simulink model "NN_EKF_Quadrotor_trajectory_control_p"  (Simulink 10.0)
settings: Solver=ode4  StartTime=0.0  StopTime=25  FixedStep=0.001  RelTol=1e-3  EnableMultiTasking=on
settings Model: Creator=Alireza  LastModifiedBy=7385281
settings DataIOCC: LimitDataPoints=on  SignalLoggingSaveFormat=ModelDataLogs
settings OptimizationCC: ExpressionDepthLimit=2147483647
settings DebuggingCC: SolverPrmCheckMsg=warning  FcnCallInpInsideContextMsg=warning  AllowSymbolicDim=off  StateNameClashWarn=warning
settings GRTTargetCC: GeneratePreprocessorConditionals=Disable all
settings ConfigComp: CovExternalEMLEnable=off

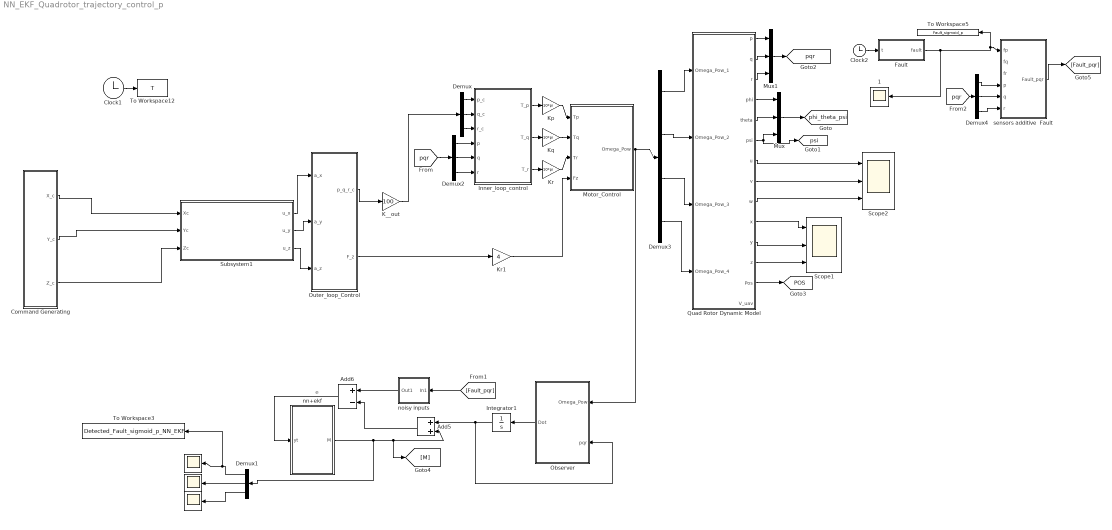
== system NN_EKF_Quadrotor_trajectory_control_p ==
  note: e
  "     " : Scope
  "      " : Scope
  "          " : Scope
  "     1" : Scope
  Add5 : Sum
  Add6 : Sum  Inputs=+-  OutDataTypeStr=Inherit: Same as accumulator
  Clock1 : Clock
  Clock2 : Clock
  Command Generating : Subsystem
  Demux{,1..2,4} (4 alike) : Demux  Outputs=3
  Demux3 : Demux
  Fault : MATLAB Function  TreatAsAtomicUnit=on
  Inner_loop_control : MATLAB Function  TreatAsAtomicUnit=on
  Integrator1 : Integrator  InitialCondition=[0.0001;0.0001;0.0001]
  K__out : Gain  Gain=100
  Kp : Gain  Gain=10*pi
  Kq : Gain  Gain=10*pi
  Kr : Gain  Gain=10*pi
  Kr1 : Gain  Gain=4
  Motor_Control : MATLAB Function  TreatAsAtomicUnit=on
  Mux : Mux  Inputs=3
  Mux1 : Mux  Inputs=3
  Observer : MATLAB Function  TreatAsAtomicUnit=on
  Outer_loop_Control : Subsystem
  Quad Rotor Dynamic Model : Subsystem
  Scope1 : Scope  NumInputPorts=3
  Scope2 : Scope  NumInputPorts=3
  Subsystem1 : Subsystem
  To Workspace12 : ToWorkspace  VariableName=T  SampleTime=-1
  To Workspace3 : ToWorkspace  VariableName=Detected_Fault_sigmoid_p_NN_EKF  SampleTime=-1
  To Workspace5 : ToWorkspace  VariableName=Fault_sigmoid_p  SampleTime=-1
  nn+ekf : Subsystem
  noisy inputs : Subsystem
  "sensors additive  Fault " : MATLAB Function  TreatAsAtomicUnit=on
  tag scope: POS=global, phi_theta_psi=global, pqr=global, psi=global
  wires:
  Quad Rotor Dynamic Model/4(phi) -> Mux/1
  Quad Rotor Dynamic Model/5(theta) -> Mux/2
  Quad Rotor Dynamic Model/6(psi) -> Mux/3, [psi]
  Mux/1 -> [phi_theta_psi]
  Inner_loop_control/1(T_p) -> Kp/1
  Inner_loop_control/2(T_q) -> Kq/1
  Inner_loop_control/3(T_r) -> Kr/1
  Quad Rotor Dynamic Model/1(p) -> Mux1/1
  Quad Rotor Dynamic Model/2(q) -> Mux1/2
  Quad Rotor Dynamic Model/3(r) -> Mux1/3
  Mux1/1 -> [pqr]
  Demux2/1 -> Inner_loop_control/4(p)
  Demux2/2 -> Inner_loop_control/5(q)
  Demux2/3 -> Inner_loop_control/6(r)
  [pqr] -> Demux2/1
  K__out/1 -> Demux/1
  Demux/1 -> Inner_loop_control/1(p_c)
  Demux/2 -> Inner_loop_control/2(q_c)
  Demux/3 -> Inner_loop_control/3(r_c)
  Quad Rotor Dynamic Model/10(x) -> Scope1/1
  Quad Rotor Dynamic Model/11(y) -> Scope1/2
  Quad Rotor Dynamic Model/12(z) -> Scope1/3
  Quad Rotor Dynamic Model/7(u) -> Scope2/1
  Quad Rotor Dynamic Model/8(v) -> Scope2/2
  Quad Rotor Dynamic Model/9(w) -> Scope2/3
  Quad Rotor Dynamic Model/13(Pos) -> [POS]
  Motor_Control/1(Omega_Pow) -> Demux3/1, Observer/1(Omega_Pow)
  Demux3/1 -> Quad Rotor Dynamic Model/1(Omega_Pow_1)
  Demux3/3 -> Quad Rotor Dynamic Model/3(Omega_Pow_3)
  Demux3/4 -> Quad Rotor Dynamic Model/4(Omega_Pow_4)
  Kp/1 -> Motor_Control/1(Tp)
  Kq/1 -> Motor_Control/2(Tq)
  Kr/1 -> Motor_Control/3(Tr)
  Demux3/2 -> Quad Rotor Dynamic Model/2(Omega_Pow_2)
  Command Generating/1(X_c) -> Subsystem1/1(Xc)
  Command Generating/2(Y_c) -> Subsystem1/2(Yc)
  Command Generating/3(Z_c) -> Subsystem1/3(Zc)
  Clock1/1 -> To Workspace12/1
  Subsystem1/1(u_x) -> Outer_loop_Control/1(a_x)
  Subsystem1/2(u_y) -> Outer_loop_Control/2(a_y)
  Subsystem1/3(u_z) -> Outer_loop_Control/3(a_z)
  Outer_loop_Control/1(p_q_r_c) -> K__out/1
  Outer_loop_Control/2(F_z) -> Kr1/1
  Kr1/1 -> Motor_Control/4(Fz)
  "sensors additive  Fault "/1(Fault_pqr) -> [Fault_pqr]
  Fault/1(fault) -> To Workspace5/1, "sensors additive  Fault "/1(fp), "     1"/1
  Observer/1(Dot) -> Integrator1/1
  Integrator1/1 -> Add5/1, Observer/2(pqr)
  Add5/1 -> Add6/2
  Add6/1 -> nn+ekf/1(yt)
  nn+ekf/1(M) -> Add5/2, [M], Demux1/1
  Demux1/3 -> "          "/1
  Demux1/1 -> "     "/1, To Workspace3/1
  Demux1/2 -> "      "/1
  [Fault_pqr] -> noisy inputs/1(In1)
  noisy inputs/1(Out1) -> Add6/1
  [pqr] -> Demux4/1
  Demux4/3 -> "sensors additive  Fault "/6(r)
  Demux4/2 -> "sensors additive  Fault "/5(q)
  Demux4/1 -> "sensors additive  Fault "/4(p)
  Clock2/1 -> Fault/1(t)

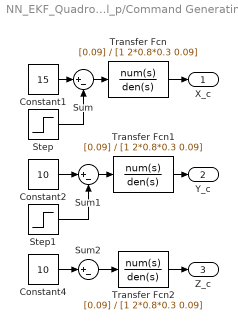
== system NN_EKF_Quadrotor_trajectory_control_p/Command Generating ==
  Constant1 : Constant  Value=15
  Constant2 : Constant  Value=10
  Constant4 : Constant  Value=10
  Step : Step  Time=30  After=15  SampleTime=0
  Step1 : Step  Time=15  After=10  SampleTime=0
  Sum : Sum  Inputs=|+-
  Sum1 : Sum  Inputs=|+-
  Sum2 : Sum  Inputs=|+-
  Transfer Fcn : TransferFcn  Numerator=[0.09]  Denominator=[1 2*0.8*0.3 0.09]
  Transfer Fcn1 : TransferFcn  Numerator=[0.09]  Denominator=[1 2*0.8*0.3 0.09]
  Transfer Fcn2 : TransferFcn  Numerator=[0.09]  Denominator=[1 2*0.8*0.3 0.09]
  X_c : Outport  VectorParamsAs1DForOutWhenUnconnected=off
  Y_c : Outport  Port=2  VectorParamsAs1DForOutWhenUnconnected=off
  Z_c : Outport  Port=3  VectorParamsAs1DForOutWhenUnconnected=off
  wires:
  Constant4/1 -> Sum2/1
  Transfer Fcn1/1 -> Y_c/1
  Transfer Fcn/1 -> X_c/1
  Constant2/1 -> Sum1/1
  Constant1/1 -> Sum/1
  Step/1 -> Sum/2
  Sum/1 -> Transfer Fcn/1
  Sum1/1 -> Transfer Fcn1/1
  Sum2/1 -> Transfer Fcn2/1
  Step1/1 -> Sum1/2
  Transfer Fcn2/1 -> Z_c/1

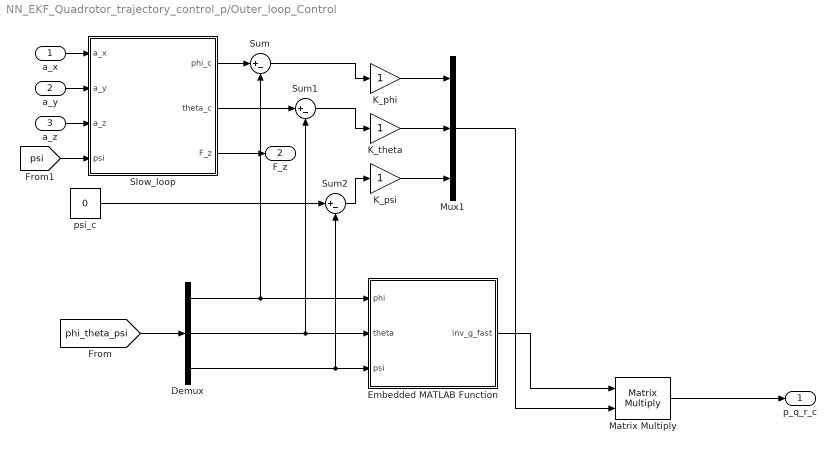
== system NN_EKF_Quadrotor_trajectory_control_p/Outer_loop_Control ==
  a_x : Inport
  a_y : Inport  Port=2
  a_z : Inport  Port=3
  Demux : Demux  Outputs=3
  Embedded MATLAB Function : MATLAB Function  TreatAsAtomicUnit=on
  K_phi : Gain
  K_psi : Gain
  K_theta : Gain
  Matrix Multiply : Product  Multiplication=Matrix(*)
  Mux1 : Mux  Inputs=3
  Slow_loop : MATLAB Function  TreatAsAtomicUnit=on
  Sum : Sum  Inputs=|+-
  Sum1 : Sum  Inputs=|+-
  Sum2 : Sum  Inputs=|+-
  psi_c : Constant  Value=0
  p_q_r_c : Outport  VectorParamsAs1DForOutWhenUnconnected=off
  F_z : Outport  Port=2  VectorParamsAs1DForOutWhenUnconnected=off
  wires:
  Sum1/1 -> K_theta/1
  Slow_loop/2(theta_c) -> Sum1/1
  Sum/1 -> K_phi/1
  Slow_loop/1(phi_c) -> Sum/1
  [phi_theta_psi] -> Demux/1
  Demux/1 -> Embedded MATLAB Function/1(phi), Sum/2
  Demux/2 -> Embedded MATLAB Function/2(theta), Sum1/2
  Demux/3 -> Embedded MATLAB Function/3(psi), Sum2/2
  psi_c/1 -> Sum2/1
  Sum2/1 -> K_psi/1
  [psi] -> Slow_loop/4(psi)
  K_phi/1 -> Mux1/1
  K_theta/1 -> Mux1/2
  K_psi/1 -> Mux1/3
  a_x/1 -> Slow_loop/1(a_x)
  a_y/1 -> Slow_loop/2(a_y)
  a_z/1 -> Slow_loop/3(a_z)
  Mux1/1 -> Matrix Multiply/2
  Slow_loop/3(F_z) -> F_z/1
  Embedded MATLAB Function/1(inv_g_fast) -> Matrix Multiply/1
  Matrix Multiply/1 -> p_q_r_c/1

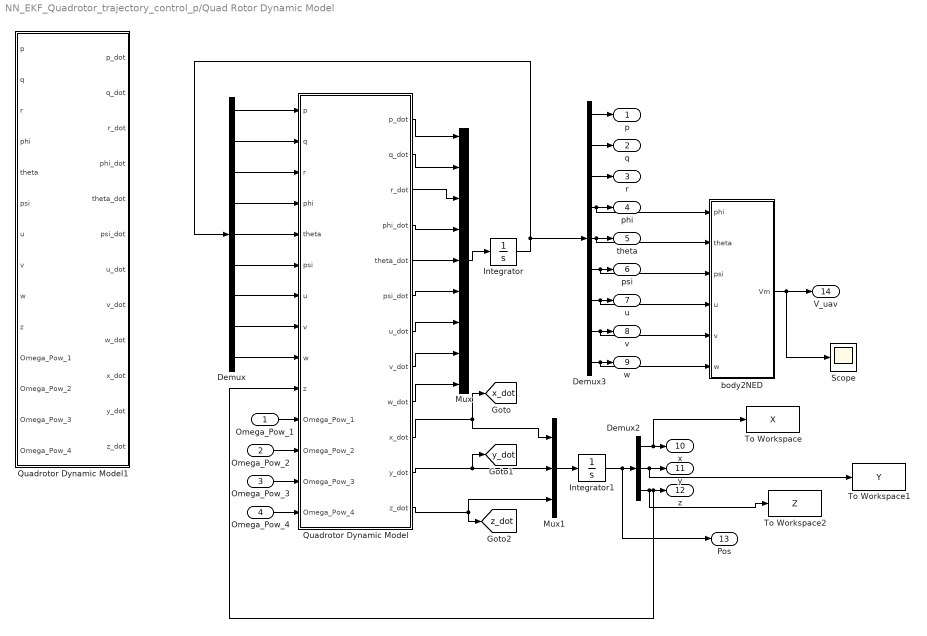
== system NN_EKF_Quadrotor_trajectory_control_p/Quad Rotor Dynamic Model ==
  Omega_Pow_1 : Inport
  Omega_Pow_2 : Inport  Port=2
  Omega_Pow_3 : Inport  Port=3
  Omega_Pow_4 : Inport  Port=4
  Demux : Demux  Outputs=9
  Demux2 : Demux  Outputs=3
  Demux3 : Demux  Outputs=9
  Integrator : Integrator  InitialCondition=[0.0001;0.0001;0.0001;0.00001;0.0001;0.0001;0.0001;0.0001;0.0001]
  Integrator1 : Integrator
  Mux : Mux  Inputs=9
  Mux1 : Mux  Inputs=3
  Quadrotor Dynamic Model : MATLAB Function  TreatAsAtomicUnit=on
  Quadrotor Dynamic Model1 : MATLAB Function  TreatAsAtomicUnit=on
  Scope : Scope
  To Workspace : ToWorkspace  VariableName=X  SampleTime=-1
  To Workspace1 : ToWorkspace  VariableName=Y  SampleTime=-1
  To Workspace2 : ToWorkspace  VariableName=Z  SampleTime=-1
  body2NED : MATLAB Function  TreatAsAtomicUnit=on
  p : Outport  VectorParamsAs1DForOutWhenUnconnected=off
  q : Outport  Port=2  VectorParamsAs1DForOutWhenUnconnected=off
  r : Outport  Port=3  VectorParamsAs1DForOutWhenUnconnected=off
  phi : Outport  Port=4  VectorParamsAs1DForOutWhenUnconnected=off
  theta : Outport  Port=5  VectorParamsAs1DForOutWhenUnconnected=off
  psi : Outport  Port=6  VectorParamsAs1DForOutWhenUnconnected=off
  u : Outport  Port=7  VectorParamsAs1DForOutWhenUnconnected=off
  v : Outport  Port=8  VectorParamsAs1DForOutWhenUnconnected=off
  w : Outport  Port=9  VectorParamsAs1DForOutWhenUnconnected=off
  x : Outport  Port=10  VectorParamsAs1DForOutWhenUnconnected=off
  y : Outport  Port=11  VectorParamsAs1DForOutWhenUnconnected=off
  z : Outport  Port=12  VectorParamsAs1DForOutWhenUnconnected=off
  Pos : Outport  Port=13  VectorParamsAs1DForOutWhenUnconnected=off
  V_uav : Outport  Port=14  VectorParamsAs1DForOutWhenUnconnected=off
  tag scope: x_dot=global, y_dot=global, z_dot=global
  wires:
  Quadrotor Dynamic Model/1(p_dot) -> Mux/1
  Quadrotor Dynamic Model/2(q_dot) -> Mux/2
  Quadrotor Dynamic Model/3(r_dot) -> Mux/3
  Quadrotor Dynamic Model/4(phi_dot) -> Mux/4
  Quadrotor Dynamic Model/5(theta_dot) -> Mux/5
  Quadrotor Dynamic Model/6(psi_dot) -> Mux/6
  Quadrotor Dynamic Model/7(u_dot) -> Mux/7
  Quadrotor Dynamic Model/8(v_dot) -> Mux/8
  Quadrotor Dynamic Model/9(w_dot) -> Mux/9
  Mux/1 -> Integrator/1
  Demux/1 -> Quadrotor Dynamic Model/1(p)
  Demux/2 -> Quadrotor Dynamic Model/2(q)
  Demux/3 -> Quadrotor Dynamic Model/3(r)
  Demux/4 -> Quadrotor Dynamic Model/4(phi)
  Demux/5 -> Quadrotor Dynamic Model/5(theta)
  Demux/6 -> Quadrotor Dynamic Model/6(psi)
  Demux/7 -> Quadrotor Dynamic Model/7(u)
  Demux/8 -> Quadrotor Dynamic Model/8(v)
  Demux/9 -> Quadrotor Dynamic Model/9(w)
  Integrator/1 -> Demux/1, Demux3/1
  Quadrotor Dynamic Model/10(x_dot) -> [x_dot], Mux1/1
  Quadrotor Dynamic Model/11(y_dot) -> Mux1/2, [y_dot]
  Quadrotor Dynamic Model/12(z_dot) -> [z_dot], Mux1/3
  Mux1/1 -> Integrator1/1
  Integrator1/1 -> Demux2/1, Pos/1
  Demux3/1 -> p/1
  Demux3/2 -> q/1
  Demux3/3 -> r/1
  Demux3/4 -> phi/1, body2NED/1(phi)
  Demux3/5 -> theta/1, body2NED/2(theta)
  Demux3/6 -> psi/1, body2NED/3(psi)
  Demux3/7 -> u/1, body2NED/4(u)
  Demux3/8 -> v/1, body2NED/5(v)
  Demux3/9 -> w/1, body2NED/6(w)
  Omega_Pow_1/1 -> Quadrotor Dynamic Model/11(Omega_Pow_1)
  Demux2/1 -> x/1, To Workspace/1
  Demux2/2 -> y/1, To Workspace1/1
  Omega_Pow_2/1 -> Quadrotor Dynamic Model/12(Omega_Pow_2)
  Demux2/3 -> z/1, Quadrotor Dynamic Model/10(z), To Workspace2/1
  Omega_Pow_3/1 -> Quadrotor Dynamic Model/13(Omega_Pow_3)
  Omega_Pow_4/1 -> Quadrotor Dynamic Model/14(Omega_Pow_4)
  body2NED/1(Vm) -> V_uav/1, Scope/1

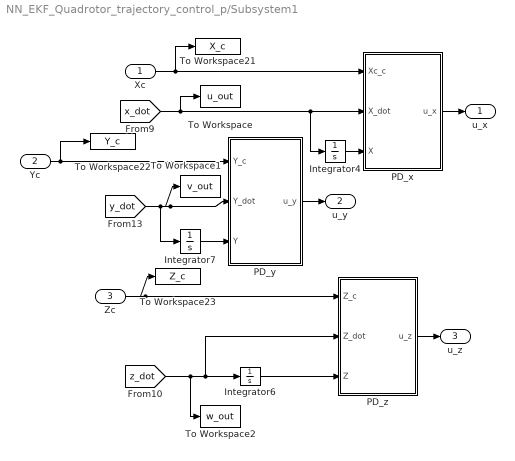
== system NN_EKF_Quadrotor_trajectory_control_p/Subsystem1 ==
  Xc : Inport
  Yc : Inport  Port=2
  Zc : Inport  Port=3
  Integrator4 : Integrator
  Integrator6 : Integrator
  Integrator7 : Integrator
  PD_x : Subsystem
  PD_y : Subsystem
  PD_z : Subsystem
  To Workspace : ToWorkspace  VariableName=u_out  SampleTime=-1
  To Workspace1 : ToWorkspace  VariableName=v_out  SampleTime=-1
  To Workspace2 : ToWorkspace  VariableName=w_out  SampleTime=-1
  To Workspace21 : ToWorkspace  VariableName=X_c  SampleTime=-1
  To Workspace22 : ToWorkspace  VariableName=Y_c  SampleTime=-1
  To Workspace23 : ToWorkspace  VariableName=Z_c  SampleTime=-1
  u_x : Outport  VectorParamsAs1DForOutWhenUnconnected=off
  u_y : Outport  Port=2  VectorParamsAs1DForOutWhenUnconnected=off
  u_z : Outport  Port=3  VectorParamsAs1DForOutWhenUnconnected=off
  wires:
  PD_z/1(u_z) -> u_z/1
  PD_y/1(u_y) -> u_y/1
  PD_x/1(u_x) -> u_x/1
  Zc/1 -> PD_z/1(Z_c), To Workspace23/1
  Yc/1 -> To Workspace22/1, PD_y/1(Y_c)
  Xc/1 -> PD_x/1(Xc_c), To Workspace21/1
  Integrator7/1 -> PD_y/3(Y)
  [x_dot] -> To Workspace/1, Integrator4/1, PD_x/2(X_dot)
  Integrator4/1 -> PD_x/3(X)
  [y_dot] -> To Workspace1/1, PD_y/2(Y_dot), Integrator7/1
  [z_dot] -> To Workspace2/1, Integrator6/1, PD_z/2(Z_dot)
  Integrator6/1 -> PD_z/3(Z)

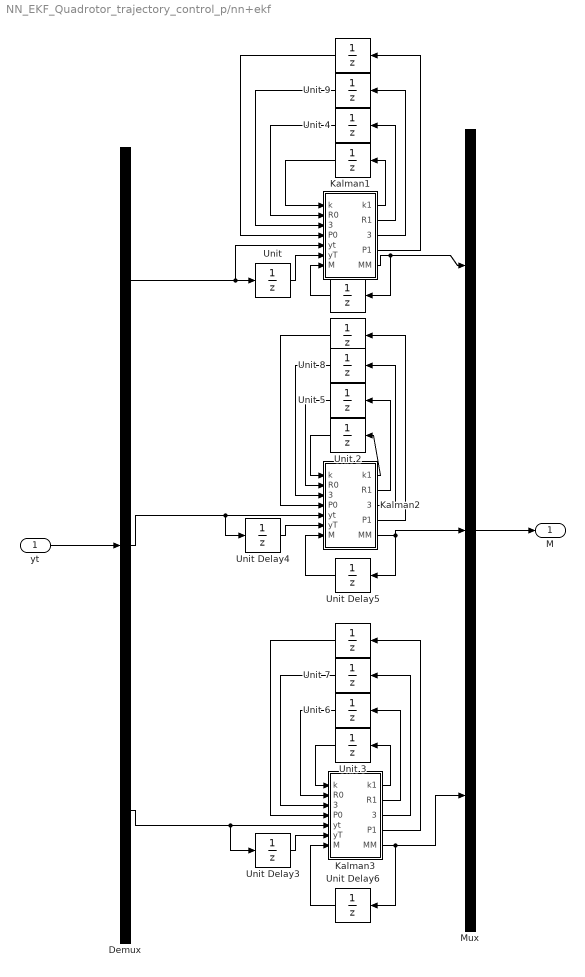
== system NN_EKF_Quadrotor_trajectory_control_p/nn+ekf ==
  yt : Inport
  " " : UnitDelay  InitialCondition=1  SampleTime=-1  HasFrameUpgradeWarning=on
  "  " : UnitDelay  InitialCondition=5*eye(3)  SampleTime=-1  HasFrameUpgradeWarning=on
  "   " : UnitDelay  InitialCondition=5*eye(3)  SampleTime=-1  HasFrameUpgradeWarning=on
  "      " : UnitDelay  InitialCondition=.01  SampleTime=-1  HasFrameUpgradeWarning=on
  "                " : UnitDelay  InitialCondition=10*eye(3)  SampleTime=-1  HasFrameUpgradeWarning=on
  Demux : Demux  Outputs=3
  Kalman1 : MATLAB Function  TreatAsAtomicUnit=on
  Kalman2 : MATLAB Function  TreatAsAtomicUnit=on
  Kalman3 : MATLAB Function  TreatAsAtomicUnit=on
  Mux : Mux  Inputs=3
  "Unit " : UnitDelay  SampleTime=-1  HasFrameUpgradeWarning=on
  Unit 2 : UnitDelay  InitialCondition=1  SampleTime=-1  HasFrameUpgradeWarning=on
  Unit 3 : UnitDelay  InitialCondition=1  SampleTime=-1  HasFrameUpgradeWarning=on
  Unit 4 : UnitDelay  InitialCondition=.00002  SampleTime=-1  HasFrameUpgradeWarning=on
  Unit 5 : UnitDelay  InitialCondition=.00002  SampleTime=-1  HasFrameUpgradeWarning=on
  Unit 6 : UnitDelay  InitialCondition=.00002  SampleTime=-1  HasFrameUpgradeWarning=on
  Unit 7 : UnitDelay  InitialCondition=[1;1;1]  SampleTime=-1  HasFrameUpgradeWarning=on
  Unit 8 : UnitDelay  InitialCondition=[1;.5;.5]  SampleTime=-1  HasFrameUpgradeWarning=on
  Unit 9 : UnitDelay  InitialCondition=[1;.5;.5]  SampleTime=-1  HasFrameUpgradeWarning=on
  Unit Delay3 : UnitDelay  SampleTime=-1  HasFrameUpgradeWarning=on
  Unit Delay4 : UnitDelay  SampleTime=-1  HasFrameUpgradeWarning=on
  Unit Delay5 : UnitDelay  InitialCondition=.01  SampleTime=-1  HasFrameUpgradeWarning=on
  Unit Delay6 : UnitDelay  InitialCondition=.01  SampleTime=-1  HasFrameUpgradeWarning=on
  M : Outport  VectorParamsAs1DForOutWhenUnconnected=off
  wires:
  "                "/1 -> Kalman3/4(P0)
  Kalman3/4(P1) -> "                "/1
  "   "/1 -> Kalman2/4(P0)
  Kalman2/4(P1) -> "   "/1
  Unit 8/1 -> Kalman2/3(teta0)
  Kalman2/3(teta1) -> Unit 8/1
  Unit 7/1 -> Kalman3/3(teta0)
  Kalman3/3(teta1) -> Unit 7/1
  Unit 6/1 -> Kalman3/2(R0)
  Kalman3/2(R1) -> Unit 6/1
  Unit 5/1 -> Kalman2/2(R0)
  Kalman2/2(R1) -> Unit 5/1
  Unit 3/1 -> Kalman3/1(k)
  Kalman3/1(k1) -> Unit 3/1
  Unit 2/1 -> Kalman2/1(k)
  Kalman2/1(k1) -> Unit 2/1
  Kalman3/5(MM) -> Unit Delay6/1, Mux/3
  Unit Delay5/1 -> Kalman2/7(M)
  Unit Delay4/1 -> Kalman2/6(yT)
  Unit Delay6/1 -> Kalman3/7(M)
  Unit Delay3/1 -> Kalman3/6(yT)
  Demux/2 -> Kalman2/5(yt), Unit Delay4/1
  Kalman2/5(MM) -> Unit Delay5/1, Mux/2
  Demux/3 -> Kalman3/5(yt), Unit Delay3/1
  Mux/1 -> M/1
  yt/1 -> Demux/1
  "  "/1 -> Kalman1/4(P0)
  Kalman1/4(P1) -> "  "/1
  Unit 9/1 -> Kalman1/3(teta0)
  Kalman1/3(teta1) -> Unit 9/1
  Unit 4/1 -> Kalman1/2(R0)
  Kalman1/2(R1) -> Unit 4/1
  " "/1 -> Kalman1/1(k)
  Kalman1/1(k1) -> " "/1
  "      "/1 -> Kalman1/7(M)
  "Unit "/1 -> Kalman1/6(yT)
  Demux/1 -> Kalman1/5(yt), "Unit "/1
  Kalman1/5(MM) -> "      "/1, Mux/1

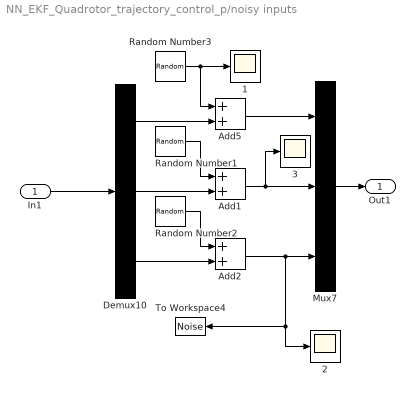
== system NN_EKF_Quadrotor_trajectory_control_p/noisy inputs ==
  In1 : Inport
  "     1" : Scope
  "     2" : Scope
  "     3" : Scope
  Add1 : Sum
  Add2 : Sum
  Add5 : Sum
  Demux10 : Demux  Outputs=3
  Mux7 : Mux  Inputs=3
  Random Number1 : RandomNumber  Variance=(1*pi/180)^2  Seed=18
  Random Number2 : RandomNumber  Variance=(1*pi/180)^2  Seed=40
  Random Number3 : RandomNumber  Variance=(1*pi/180)^2  Seed=68
  To Workspace4 : ToWorkspace  VariableName=Noise  SampleTime=-1
  Out1 : Outport  VectorParamsAs1DForOutWhenUnconnected=off
  wires:
  In1/1 -> Demux10/1
  Mux7/1 -> Out1/1
  Random Number3/1 -> Add5/1, "     1"/1
  Demux10/1 -> Add5/2
  Add5/1 -> Mux7/1
  Random Number1/1 -> Add1/1
  Demux10/2 -> Add1/2
  Add1/1 -> Mux7/2, "     3"/1
  Random Number2/1 -> Add2/1
  Demux10/3 -> Add2/2
  Add2/1 -> Mux7/3, "     2"/1, To Workspace4/1

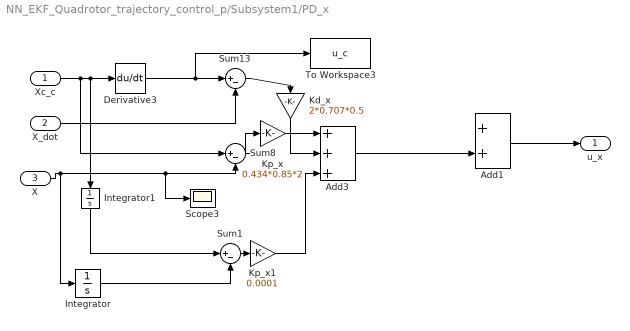
== system NN_EKF_Quadrotor_trajectory_control_p/Subsystem1/PD_x ==
  Xc_c : Inport
  X_dot : Inport  Port=2
  X : Inport  Port=3
  Add1 : Sum
  Add3 : Sum  Inputs=+++
  Derivative3 : Derivative
  Integrator : Integrator
  Integrator1 : Integrator
  Kd_x : Gain  Gain=2*0.707*0.5
  Kp_x : Gain  Gain=0.434*0.85*2
  Kp_x1 : Gain  Gain=0.0001
  Scope3 : Scope
  Sum1 : Sum  Inputs=|+-
  Sum13 : Sum  Inputs=|+-
  Sum8 : Sum  Inputs=|+-
  To Workspace3 : ToWorkspace  VariableName=u_c  SampleTime=-1
  u_x : Outport  VectorParamsAs1DForOutWhenUnconnected=off
  wires:
  Add3/1 -> Add1/2
  Add1/1 -> u_x/1
  Kp_x1/1 -> Add3/3
  Integrator1/1 -> Sum1/1
  Integrator/1 -> Sum1/2
  Sum1/1 -> Kp_x1/1
  X_dot/1 -> Sum13/2
  Xc_c/1 -> Integrator1/1, Derivative3/1, Sum8/1
  Kp_x/1 -> Add3/2
  Kd_x/1 -> Add3/1
  Sum13/1 -> Kd_x/1
  Derivative3/1 -> To Workspace3/1, Sum13/1
  X/1 -> Integrator/1, Sum8/2, Scope3/1
  Sum8/1 -> Kp_x/1

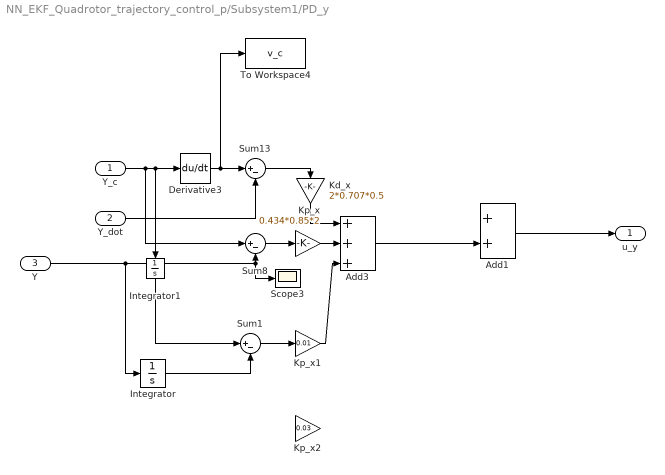
== system NN_EKF_Quadrotor_trajectory_control_p/Subsystem1/PD_y ==
  Y_c : Inport
  Y_dot : Inport  Port=2
  Y : Inport  Port=3
  Add1 : Sum
  Add3 : Sum  Inputs=+++
  Derivative3 : Derivative
  Integrator : Integrator
  Integrator1 : Integrator
  Kd_x : Gain  Gain=2*0.707*0.5
  Kp_x : Gain  Gain=0.434*0.85*2
  Kp_x1 : Gain  Gain=0.01
  Kp_x2 : Gain  Gain=0.03
  Scope3 : Scope
  Sum1 : Sum  Inputs=|+-
  Sum13 : Sum  Inputs=|+-
  Sum8 : Sum  Inputs=|+-
  To Workspace4 : ToWorkspace  VariableName=v_c  SampleTime=-1
  u_y : Outport  VectorParamsAs1DForOutWhenUnconnected=off
  wires:
  Add1/1 -> u_y/1
  Add3/1 -> Add1/2
  Y_dot/1 -> Sum13/2
  Y_c/1 -> Integrator1/1, Derivative3/1, Sum8/1
  Kp_x1/1 -> Add3/3
  Integrator1/1 -> Sum1/1
  Integrator/1 -> Sum1/2
  Sum1/1 -> Kp_x1/1
  Kp_x/1 -> Add3/2
  Kd_x/1 -> Add3/1
  Sum13/1 -> Kd_x/1
  Derivative3/1 -> Sum13/1, To Workspace4/1
  Y/1 -> Integrator/1, Sum8/2, Scope3/1
  Sum8/1 -> Kp_x/1

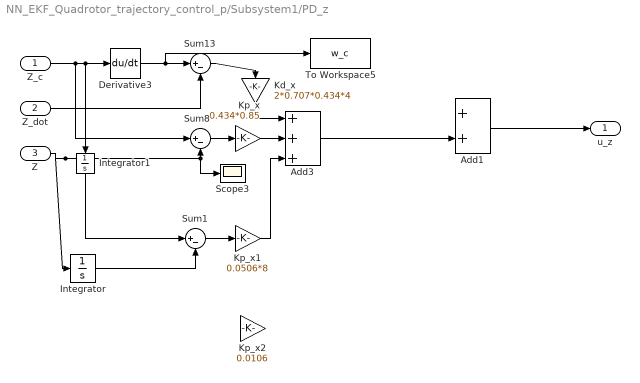
== system NN_EKF_Quadrotor_trajectory_control_p/Subsystem1/PD_z ==
  Z_c : Inport
  Z_dot : Inport  Port=2
  Z : Inport  Port=3
  Add1 : Sum
  Add3 : Sum  Inputs=+++
  Derivative3 : Derivative
  Integrator : Integrator
  Integrator1 : Integrator
  Kd_x : Gain  Gain=2*0.707*0.434*4
  Kp_x : Gain  Gain=0.434*0.85
  Kp_x1 : Gain  Gain=0.0506*8
  Kp_x2 : Gain  Gain=0.0106
  Scope3 : Scope
  Sum1 : Sum  Inputs=|+-
  Sum13 : Sum  Inputs=|+-
  Sum8 : Sum  Inputs=|+-
  To Workspace5 : ToWorkspace  VariableName=w_c  SampleTime=-1
  u_z : Outport  VectorParamsAs1DForOutWhenUnconnected=off
  wires:
  Add3/1 -> Add1/2
  Add1/1 -> u_z/1
  Z_dot/1 -> Sum13/2
  Z_c/1 -> Integrator1/1, Derivative3/1, Sum8/1
  Kp_x1/1 -> Add3/3
  Integrator1/1 -> Sum1/1
  Integrator/1 -> Sum1/2
  Sum1/1 -> Kp_x1/1
  Kp_x/1 -> Add3/2
  Kd_x/1 -> Add3/1
  Sum13/1 -> Kd_x/1
  Derivative3/1 -> To Workspace5/1, Sum13/1
  Z/1 -> Integrator/1, Sum8/2, Scope3/1
  Sum8/1 -> Kp_x/1

== matlab function Outer_loop_Control/Embedded MATLAB Function ==
  data: phi input double; inv_g_fast output double; theta input double; psi input double
function inv_g_fast = fcn(phi,theta,psi)
g=[1 sin(phi)*tan(theta) cos(phi)*tan(theta)
    0 cos(phi) -sin(phi)
    0 sin(phi)/cos(theta) cos(phi)/cos(theta)];
inv_g_fast=inv(g);

== matlab function Quad Rotor Dynamic Model/Quadrotor Dynamic Model ==
  data: p input double; q input double; r input double; phi input double; theta input double; psi input double; u input double; p_dot output double; v input double; w input double; z input double; Omega_Pow_1 input double; Omega_Pow_2 input double; Omega_Pow_3 input double; Omega_Pow_4 input double; q_dot output double; r_dot output double; phi_dot output double; theta_dot output double; psi_dot output double; u_dot output double; v_dot output double; w_dot output double; x_dot output double; y_dot output double; z_dot output double
function [p_dot,q_dot,r_dot,phi_dot,theta_dot,psi_dot,u_dot,v_dot,w_dot,x_dot,y_dot,z_dot] = fcn(p,q,r,phi,theta,psi,u,v,w,z,...
    Omega_Pow_1,Omega_Pow_2,Omega_Pow_3,Omega_Pow_4)

%% System Parameters
g=9.81;
m=2.3; %kg (mass of quadrotor)
L=0.7; %m Lever arm
Ix=8.04*10^(-3); % kgm^2 Body of inertia of x axsis
Iy=8.46*10^(-3);%kgm^2 Body of inertia of y axsis
Iz=16.48*10^(-3);%kgm^2 Body of inertia of z axsis
K_f=0.65016e-3; %N/(rad/s)^2 Force coefficient
K_t=0.82218e-5; %N/(rad/s)^2 Torque coefficient
K1=20; % Motor Model coefficient
K2=0.01; % Motor Model coefficient
K3=3.5; % Motor Model coefficient
z_l=0.003; %m Elastic deformation of the gear
k_l=6000; % N/m Elastic Coefficient of the gear.
if (z-z_l)>0
    delta_z_l=1;
else delta_z_l=0;
end

Tp=L*K_f*(-Omega_Pow_1^2+Omega_Pow_2^2+Omega_Pow_3^2-Omega_Pow_4^2);
Tq=L*K_f*(-Omega_Pow_1^2+Omega_Pow_2^2-Omega_Pow_3^2+Omega_Pow_4^2);
Tr=L*K_t*(Omega_Pow_1^2+Omega_Pow_2^2-Omega_Pow_3^2-Omega_Pow_4^2);
Fz=K_f*(Omega_Pow_1^2+Omega_Pow_2^2+Omega_Pow_3^2+Omega_Pow_4^2);
%Quadrotor Dynamic
p_dot=(-q*r*(Iz-Iy)/Ix)+Tp/Ix;
q_dot=(-p*r*(Ix-Iz)/Iy)+Tq/Iy;
r_dot=(-p*q*(Iy-Ix)/Iz)+Tr/Iz;
%%%%%%%%%%%%%%%%%%%%%%%%%%%
phi_dot=p+sin(phi)*tan(theta)*q+cos(phi)*tan(theta)*r;
theta_dot=cos(phi)*q-sin(phi)*q;
psi_dot=(sin(phi)/cos(theta))*q+(cos(phi)/cos(theta))*r;
%%%%%%%%%%%%%%%%%%%%%%%%%%%%%%%%%%%%%%%%%
u_dot=r*v-q*w+g*sin(theta);
v_dot=-r*u+p*w-g*cos(theta)*sin(phi);
w_dot=q*u-p*v+Fz/m-g*cos(theta)*cos(phi)+K1*(z_l-z)*delta_z_l/m;
%%%%%%%%%%%%%%%%%%%%%%%%%%%%%%%%%%%%%%%%%%%%%%%%
x_dot=cos(theta)*cos(psi)*u+(-cos(phi)*sin(psi)+sin(phi)*sin(theta)*cos(psi))*v+(sin(phi)*sin(psi)+cos(phi)*sin(theta)*cos(psi))*w;
y_dot=cos(theta)*sin(psi)*u+(cos(phi)*cos(psi)+sin(phi)*sin(theta)*sin(psi))*v+(-sin(phi)*cos(psi)+cos(phi)*sin(theta)*sin(psi))*w;
z_dot=-sin(theta)*u+sin(phi)*cos(theta)*v+cos(phi)*cos(theta)*w;
%%%%%%%%%%Motor Speed Model



y = u;

== matlab function Outer_loop_Control/Slow_loop ==
  data: phi_c output double; theta_c output double; a_x input double; a_y input double; a_z input double; F_z output double; psi input double
function [phi_c,theta_c,F_z] = fcn(a_x,a_y,a_z,psi)
g=9.81;
m=2.3; %kg (mass of quadrotor)
F_z=(a_z+g)*m;
phi_c=(a_x*sin(psi)-a_y*cos(psi))*m/F_z;
theta_c=(a_x*cos(psi)+a_y*sin(psi))*m/F_z;

== matlab function Inner_loop_control ==
  data: p_c input double; T_p output double; q_c input double; T_q output double; T_r output double; r_c input double; p input double; q input double; r input double
function [T_p,T_q,T_r] = fcn(p_c,q_c,r_c,p,q,r)
Ix=8.04*10^(-3); % kgm^2 Body of inertia of x axsis
Iy=8.46*10^(-3);%kgm^2 Body of inertia of y axsis
Iz=16.48*10^(-3);%kgm^2 Body of inertia of z axsis

T_p=(p_c-p)*Ix;
T_q=(q_c-q)*Iy;
T_r=(r_c-r)*Iz;

== matlab function Motor_Control ==
  data: Tp input double; Omega_Pow output double; Tq input double; Tr input double; Fz input double
function Omega_Pow = fcn(Tp,Tq,Tr,Fz)
Kf=0.65016e-3; %N/(rad/s)^2 Force coefficient
Kt=0.82218e-5; %N/(rad/s)^2 Torque coefficient
L=0.7; %m Lever arm

Omega_Pow_2=[-0.25 -0.25 0.25 0.25;0.25 0.25 0.25 0.25; 0.25 -0.25 -0.25 0.25; -0.25 0.25 -0.25 0.25]*...
   [Tp/(L*Kf);Tq/(L*Kf);Tr/(L*Kt);Fz/Kf];
Omega_Pow=sqrt(abs(Omega_Pow_2));

== matlab function Fault ==
  data: t input double; fault output double
function fault = fcn(t)
t0=5;
omega=0.01;
if t<=t0
    fault=0;
else
    fault=1-exp(-omega*(t-t0));
end

== matlab function Observer ==
  data: Omega_Pow input double; Dot output double; pqr input double
function Dot   = fcn(Omega_Pow,pqr)
p=pqr(1);
q=pqr(2);
r=pqr(3);
Omega_Pow_1=Omega_Pow(1);
Omega_Pow_2=Omega_Pow(2);
Omega_Pow_3=Omega_Pow(3);
Omega_Pow_4=Omega_Pow(4);

% Equations Of Motion
L=0.7; %m Lever arm
Ix=8.04*10^(-3); % kgm^2 Body of inertia of x axsis
Iy=8.46*10^(-3);%kgm^2 Body of inertia of y axsis
Iz=16.48*10^(-3);%kgm^2 Body of inertia of z axsis
K_f=0.65016e-3; %N/(rad/s)^2 Force coefficient
K_t=0.82218e-5; %N/(rad/s)^2 Torque coefficient

Tp=L*K_f*(-Omega_Pow_1^2+Omega_Pow_2^2+Omega_Pow_3^2-Omega_Pow_4^2);
Tq=L*K_f*(-Omega_Pow_1^2+Omega_Pow_2^2-Omega_Pow_3^2+Omega_Pow_4^2);
Tr=L*K_t*(Omega_Pow_1^2+Omega_Pow_2^2-Omega_Pow_3^2-Omega_Pow_4^2);

%Quadrotor Dynamic
p_dot=(-q*r*(Iz-Iy)/Ix)+Tp/Ix;
q_dot=(-p*r*(Ix-Iz)/Iy)+Tq/Iy;
r_dot=(-p*q*(Iy-Ix)/Iz)+Tr/Iz;
%==============================
Dot=[p_dot;q_dot;r_dot];

== matlab function nn+ekf/Kalman1 ==
  data: k1 output double; R1 output double; teta1 output double; P1 output double; k input double; R0 input double; teta0 input double; P0 input double; MM output double; yt input double; yT input double; M input double
function [k1,R1,teta1,P1,MM]  = fcn(k,R0,teta0,P0,yt,yT,M)
eta=1.5;
Z=teta0(2)*M+teta0(3)*yT;
sigma=(1-exp(-Z))/(1+exp(-Z));
H=[sigma;teta0(1)*M*0.5*(1-sigma^2);teta0(1)*yT*0.5*(1-sigma^2)];
R1=R0+(yt^2-R0)/k;
K=P0*H*(((H'*P0*H)+R1)^(-1));
teta1=teta0+eta*K*(yt);
n=teta1(2)*M+teta1(3)*yT;
MM=teta1(1)*((1-exp(-n))/(1+exp(-n)));
P1=P0-K*H'*P0;
k1=k+1;

== matlab function nn+ekf/Kalman2 ==
  data: k1 output double; R1 output double; teta1 output double; P1 output double; k input double; R0 input double; teta0 input double; P0 input double; MM output double; yt input double; yT input double; M input double
function [k1,R1,teta1,P1,MM]  = fcn(k,R0,teta0,P0,yt,yT,M)
eta=1;
Z=teta0(2)*M+teta0(3)*yT;
sigma=(1-exp(-Z))/(1+exp(-Z));
H=[sigma;teta0(1)*M*.5*(1-sigma^2);teta0(1)*yT*0.5*(1-sigma^2)];
R1=R0+(yt^2-R0)/k;
K=P0*H*(((H'*P0*H)+R1)^(-1));
teta1=teta0+eta*K*(yt);
n=teta1(2)*M+teta1(3)*yT;
MM=teta1(1)*((1-exp(-n))/(1+exp(-n)));
P1=P0-K*H'*P0;
k1=k+1;

== matlab function nn+ekf/Kalman3 ==
  data: k1 output double; R1 output double; teta1 output double; P1 output double; k input double; R0 input double; teta0 input double; P0 input double; MM output double; yt input double; yT input double; M input double
function [k1,R1,teta1,P1,MM] = fcn(k,R0,teta0,P0,yt,yT,M)
eta=1;
Z=teta0(2)*M+teta0(3)*yT;
sigma=(1-exp(-Z))/(1+exp(-Z));
H=[sigma;teta0(1)*M*0.5*(1-sigma^2);teta0(1)*yT*0.5*(1-sigma^2)];
R1=R0+(yt^2-R0)/k;
K=P0*H*(((H'*P0*H)+R1)^(-1));
teta1=teta0+eta*K*(yt);
n=teta1(2)*M+teta1(3)*yT;
MM=teta1(1)*((1-exp(-n))/(1+exp(-n)));
P1=P0-K*H'*P0;
k1=k+1;

== matlab function Quad Rotor Dynamic Model/body2NED ==
  data: phi input double; theta input double; psi input double; u input double; v input double; w input double; Vm output double
function Vm= fcn(phi,theta,psi,u,v,w)
N=[cos(theta)*cos(psi) (sin(phi)*sin(theta)*cos(psi)-cos(phi)*sin(psi)) (cos(phi)*sin(theta)*cos(psi)+sin(phi)*sin(psi));
   -cos(theta)*sin(psi) -(sin(phi)*sin(theta)*sin(psi)+cos(phi)*cos(psi)) -(cos(phi)*sin(theta)*sin(psi) - sin(phi)*cos(psi));
   sin(theta) -sin(phi)*cos(theta) -cos(phi)*cos(theta)];
Vm=N*[u;v;w];
end

== matlab function Quad Rotor Dynamic Model/Quadrotor Dynamic Model1 ==
  data: p input double; q input double; r input double; phi input double; theta input double; psi input double; u input double; p_dot output double; v input double; w input double; z input double; Omega_Pow_1 input double; Omega_Pow_2 input double; Omega_Pow_3 input double; Omega_Pow_4 input double; q_dot output double; r_dot output double; phi_dot output double; theta_dot output double; psi_dot output double; u_dot output double; v_dot output double; w_dot output double; x_dot output double; y_dot output double; z_dot output double
function [p_dot,q_dot,r_dot,phi_dot,theta_dot,psi_dot,u_dot,v_dot,w_dot,x_dot,y_dot,z_dot] = fcn(p,q,r,phi,theta,psi,u,v,w,z,...
    Omega_Pow_1,Omega_Pow_2,Omega_Pow_3,Omega_Pow_4)

%% System Parameters
g=9.81;
m=2.3; %kg (mass of quadrotor)
L=0.7; %m Lever arm
Ix=8.04*10^(-3); % kgm^2 Body of inertia of x axsis
Iy=8.46*10^(-3);%kgm^2 Body of inertia of y axsis
Iz=16.48*10^(-3);%kgm^2 Body of inertia of z axsis
K_f=0.65016e-3; %N/(rad/s)^2 Force coefficient
K_t=0.82218e-5; %N/(rad/s)^2 Torque coefficient
K1=20; % Motor Model coefficient
K2=0.01; % Motor Model coefficient
K3=3.5; % Motor Model coefficient
z_l=0.003; %m Elastic deformation of the gear
k_l=6000; % N/m Elastic Coefficient of the gear.
if (z-z_l)>0
    delta_z_l=1;
else delta_z_l=0;
end

Tp=L*K_f*(-Omega_Pow_1^2+Omega_Pow_2^2+Omega_Pow_3^2-Omega_Pow_4^2);
Tq=L*K_f*(-Omega_Pow_1^2+Omega_Pow_2^2-Omega_Pow_3^2+Omega_Pow_4^2);
Tr=L*K_t*(Omega_Pow_1^2+Omega_Pow_2^2-Omega_Pow_3^2-Omega_Pow_4^2);
Fz=K_f*(Omega_Pow_1^2+Omega_Pow_2^2+Omega_Pow_3^2+Omega_Pow_4^2);
%Quadrotor Dynamic
p_dot=(-q*r*(Iz-Iy)/Ix)+Tp/Ix;
q_dot=(-p*r*(Ix-Iz)/Iy)+Tq/Iy;
r_dot=(-p*q*(Iy-Ix)/Iz)+Tr/Iz;
%%%%%%%%%%%%%%%%%%%%%%%%%%%
phi_dot=p+sin(phi)*tan(theta)*q+cos(phi)*tan(theta)*r;
theta_dot=cos(phi)*q-sin(phi)*q;
psi_dot=(sin(phi)/cos(theta))*q+(cos(phi)/cos(theta))*r;
%%%%%%%%%%%%%%%%%%%%%%%%%%%%%%%%%%%%%%%%%
u_dot=r*v-q*w+g*sin(theta);
v_dot=-r*u+p*w-g*cos(theta)*sin(phi);
w_dot=q*u-p*v+Fz/m-g*cos(theta)*cos(phi)+K1*(z_l-z)*delta_z_l/m;
%%%%%%%%%%%%%%%%%%%%%%%%%%%%%%%%%%%%%%%%%%%%%%%%
x_dot=cos(theta)*cos(psi)*u+(-cos(phi)*sin(psi)+sin(phi)*sin(theta)*cos(psi))*v+(sin(phi)*sin(psi)+cos(phi)*sin(theta)*cos(psi))*w;
y_dot=cos(theta)*sin(psi)*u+(cos(phi)*cos(psi)+sin(phi)*sin(theta)*sin(psi))*v+(-sin(phi)*cos(psi)+cos(phi)*sin(theta)*sin(psi))*w;
z_dot=-sin(theta)*u+sin(phi)*cos(theta)*v+cos(phi)*cos(theta)*w;
%%%%%%%%%%Motor Speed Model



y = u;

== matlab function sensors additive  Fault  ==
  data: fp input double; Fault_pqr output double; fq input double; fr input double; p input double; q input double; r input double
function Fault_pqr = fcn(fp,fq,fr,p,q,r)

Fault_pqr = [p;q;r]+[fp;fq;fr]+[.00060;.000001;.000001];
